simulink library "fdctools"  (Simulink 3.00)
libraries: simulink3 x3
settings Model: LastModifiedBy=Dutchroll

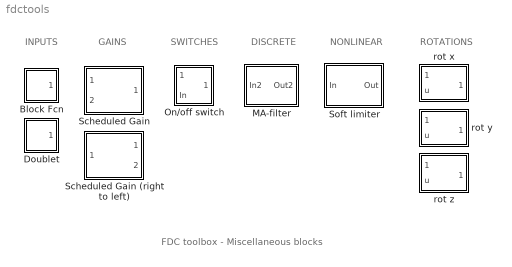
== system fdctools ==
  note: FDC toolbox - Miscellaneous blocks
  note: GAINS
  note: SWITCHES
  note: DISCRETE
  note: NONLINEAR
  note: INPUTS
  note: ROTATIONS
  Block Fcn : Subsystem  mask(Block Fcn){yinit=-1, yblock=2, tstart=1, tstop=4}
      mask prompts: yinit "Initial value (=final value):"; yblock "Amplitude of block (+ = step up, - = step down):"; tstart "Start time of block:"; tstop "Stop time of block:"
      mask help: Block Function
      mask Help:
      | This block implements a block signal.<br><br>
      | Parameters:
      | <li>the initial (=final) value of the signal,
      | <li>the amplitude of the block (positive = upwards, negative = downwards),
      | <li>the start time, and
      | <li>the stop time (which must be later than the start time).
      mask Display: plot(0,0,100,100,[100,60,60,20,20,0],[50,50,89,89,50,50])
  Doublet : Subsystem  mask(Doublet){ts1=1, dt1=1, dt2=1, y1=1, y2=-1, cnst=0}
      mask prompts: ts1 "Start time [sec]:"; dt1 "Length of time interval 1 [sec]:"; dt2 "Length of time interval 2 [sec]:"; cnst "y start (= y final):"
      mask help: Doublet signal.
      mask Help:
      | This block implements a doublet signal:<br><br>
      | y = y1 if  (tstart <= t < tstart+dt1), <br><br>
      | y = y2 if  (tstart+dt1 <= t < tstart+dt1+dt2), <br><br>
      | y = ystart = yfinal if (t < tstart) or (t > tstart+dt1+dt2).<br><br>
      | where tstart is the start time, dt1 is the length of the first time-interval and dt2 is the length of the second time-interval.
      mask Display: plot([0 1 1 2.5 2.5 4 4 5],[0 0 1 1 -1.5 -1.5 0 0])
  MA-filter : Subsystem  mask(Moving Average filter){ns=5, Ts=0.1, uinit=0}
      mask prompts: ns "Number of samples for averaging:"; Ts "Sample time:"; uinit "Initial value of input signal:"
      mask help: Digital Moving Average filter
      mask init:
      | Ama=[zeros(1,ns);[eye(ns-1) zeros(ns-1,1)]]; Bma=[1; zeros(ns-1,1)]; Cma=1/ns*ones(1,ns); Dma=0; xinit=uinit*ones(ns,1);
      mask Help:
      | Digital Moving Average filter.<br><br>
      | y(k) = 1/ns * (u(k) + u(k-1) + ... + u(k-ns)),<br><br>
      | where ns is the number of samples for averaging (to be specified by the user).
      mask Display: disp('Moving\nAverage')
  On/off switch : Subsystem
      mask Type: On/off switch
      mask Description:
      | If input(1) = 1
      |      output = input(2)
      |  else if input(1) = 0
      |      output = 0
      mask Help:
      | On/off switch. If the first input signal is equal to 1, the second input signal will be sent to the output port. Else, if the first input signal is equal to zero, the output signal will be zero.<br><br>
      | 
      | Note: for other values of the first input signal, the resulting output will be unpredictable!
      mask Display: plot(0,0,100,100,[31,31,32,34,34,32,31,31,0],[50,48,47,48,51,53,51,50,50],[100,75,51],[50,50,97]);disp('?')
  Scheduled Gain : Subsystem  mask(Scheduled Gain){K=sin(u[1])}
      mask prompts: K "Gain function:"
      mask help:
      | Inputs: u1 and u2.
      | Output: y.
      |
      | Output equation:   y = K(u1) * u2
      |
      | K is the gain-function, which must be entered below. See the description of the Fcn block from the Nonlinear library for details about valid expressions and the block-characteristics.
      mask init:
      | blockname = [gcb, '/Gain Fcn K(u1)'];
      | set_param(blockname,'Expr',K)
      mask Help:
      | Scheduled Gain function.<br><br>
      | Inputs: u1 and u2, <br><br>
      | output: y, <br><br>
      | output equation:   y = K(u1) * u2.<br><br>
      | K is the gain-function, which must be entered as block-parameter. See the description of the Fcn block from the Nonlinear library for details about valid expressions and the block-characteristics.
      mask Display: plot([0,100,0,0],[0,46,100,0]);disp('K(u1)      ');
  Scheduled Gain (right to left) : Subsystem  Orientation=left  mask(Scheduled Gain){K=sin(u[1])}
      mask prompts: K "Gain function:"
      mask help:
      | Inputs: u1 and u2.
      | Output: y.
      |
      | Output equation:   y = K(u1) * u2
      |
      | K is the gain-function, which must be entered below. See the description of the Fcn block from the Nonlinear library for details about valid expressions and the block-characteristics.
      mask init:
      | blockname = [gcb, '/Gain Fcn K(u1)'];
      | set_param(blockname,'Expr',K)
      mask Help:
      | Scheduled Gain function.<br><br>
      | Inputs: u1 and u2, <br><br>
      | output: y, <br><br>
      | output equation:   y = K(u1) * u2.<br><br>
      | K is the gain-function, which must be entered as block-parameter. See the description of the Fcn block from the Nonlinear library for details about valid expressions and the block-characteristics.
      mask Display: plot([0,-100,0,0],[0,46,100,0]);disp('        K(u1)');
  Soft limiter : Subsystem  mask(Soft limiter){@1=10, @2=10}
      mask prompts: @1 "Limiter range= max. output value= --(min. output value):"; @2 "% of output range where y=u (linear throughput):"
      mask help: Soft limiter with partly linear throughput.
      mask init:
      | max_u=max(@1,1e-16); lin_u=min(0.9999,(max(@2,0)/100))*max_u; uplot=[-5*max_u:0.25*max_u:5*max_u]; for i = 1:length(uplot); yplot(i)=softlim([],[],uplot(i),3,max_u,lin_u); end;
      mask Help:
      | Soft limiter with partly linear throughput. See the source-code of SOFTLIM.M or type HELP SOFTLIM at the command-line to see how this works.<br><br>
      | Parameters:<br><br>
      | <li>Limiter range = maximum output value, which equal <i>minus</i> the minimum output value,
      | <li>percentage of output range where y=u (in this part of the output range the function will yield a linear throughput).
      mask Display: plot(uplot, yplot, max_u*[-5,-1,1,5], max_u*[-1,-1,1,1], 0, -1.3*max_u, 0, 1.2*max_u, max_u*[-5,5], [0,0]);
  rot x : Subsystem
      mask Type: Rotation around X-axis
      mask Description: Direction cosines for rotation around positive X-axis. The first input signal is a (3x1) vector which will be converted to the new reference frame. The second input is a scalar value, which represents the rotation angle.
      mask Help:
      | Direction cosines for rotation around positive X-axis.<br><br>
      | The first input signal is a (3x1) vector which will be converted to the new reference frame. The second input is a scalar value, which represents the rotation angle.
      mask Display: disp('rot x')
  rot y : Subsystem
      mask Type: Rotation around Y-axis
      mask Description: Direction cosines for rotation around positive Y-axis. The first input signal is a (3x1) vector which will be converted to the new reference frame. The second input is a scalar value, which represents the rotation angle.
      mask Help:
      | Direction cosines for rotation around positive Y-axis.<br><br>
      |  The first input signal is a (3x1) vector which will be converted to the new reference frame. The second input is a scalar value, which represents the rotation angle.
      mask Display: disp('rot y')
  rot z : Subsystem
      mask Type: Rotation around Z-axis
      mask Description: Direction cosines for rotation around positive Z-axis. The first input signal is a (3x1) vector which will be converted to the new reference frame. The second input is a scalar value, which represents the rotation angle.
      mask Help:
      | Direction cosines for rotation around positive Z-axis.<br><br>
      | The first input signal is a (3x1) vector which will be converted to the new reference frame. The second input is a scalar value, which represents the rotation angle.
      mask Display: disp('rot z')

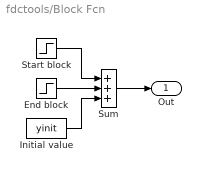
== system fdctools/Block Fcn ==
  End block : Step  Time=tstop  Before=0  After=-yblock  SampleTime=0
  Initial value : Constant  Value=yinit
  Start block : Step  Time=tstart  Before=0  After=yblock  SampleTime=0
  Sum : Sum  Inputs=+++  SaturateOnIntegerOverflow=on
  Out : Outport  Port=1
  wires:
  Initial value/1 -> Sum/3
  Start block/1 -> Sum/1
  End block/1 -> Sum/2
  Sum/1 -> Out/1

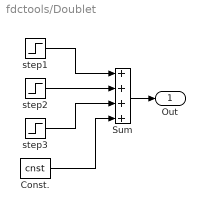
== system fdctools/Doublet ==
  Const. : Constant  Value=cnst
  Sum : Sum  Inputs=++++  SaturateOnIntegerOverflow=on
  step1 : Step  Time=ts1  Before=0  After=y1-cnst  SampleTime=0
  step2 : Step  Time=ts1+dt1  Before=0  After=-y1+y2  SampleTime=0
  step3 : Step  Time=ts1+dt1+dt2  Before=0  After=-y2+cnst  SampleTime=0
  Out : Outport  Port=1
  wires:
  Const./1 -> Sum/4
  step1/1 -> Sum/1
  step2/1 -> Sum/2
  step3/1 -> Sum/3
  Sum/1 -> Out/1

== system fdctools/MA-filter ==
  In2 : Inport  Port=1  PortWidth=-1  SampleTime=-1  DataType=auto
      settings: SignalType=auto
  MA-filter : DiscreteStateSpace  A=Ama  B=Bma  C=Cma  D=Dma  X0=xinit  SampleTime=Ts
  Out2 : Outport  Port=1
  wires:
  In2/1 -> MA-filter/1
  MA-filter/1 -> Out2/1

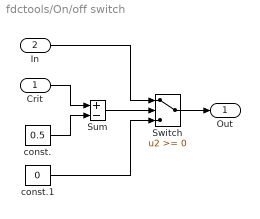
== system fdctools/On/off switch ==
  Crit : Inport  Port=1  PortWidth=-1  SampleTime=-1  DataType=auto
      settings: SignalType=auto
  In : Inport  Port=2  PortWidth=-1  SampleTime=-1  DataType=auto
      settings: SignalType=auto
  Sum : Sum  Inputs=+-  SaturateOnIntegerOverflow=on
  Switch : Switch  Threshold=0
  const. : Constant  Value=0.5
  const.1 : Constant  Value=0
  Out : Outport  Port=1
  wires:
  Crit/1 -> Sum/1
  const.1/1 -> Switch/3
  Sum/1 -> Switch/2
  Switch/1 -> Out/1
  In/1 -> Switch/1
  const./1 -> Sum/2

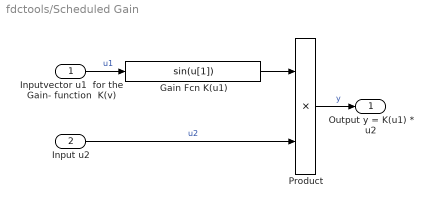
== system fdctools/Scheduled Gain ==
  Inputvector u1  for the Gain- function  K(v) : Inport  Port=1  PortWidth=-1  SampleTime=-1  DataType=auto
      settings: SignalType=auto
  Input u2 : Inport  Port=2  PortWidth=-1  SampleTime=-1  DataType=auto
      settings: SignalType=auto
  Gain Fcn K(u1) : Fcn  Expr=sin(u[1])
  Product : Product  Inputs=2  SaturateOnIntegerOverflow=on
  Output y = K(u1) * u2 : Outport  Port=1
  wires:
  Gain Fcn K(u1)/1 -> Product/1
  Input u2/1 -> Product/2  "u2"
  Product/1 -> Output y = K(u1) * u2/1  "y"
  Inputvector u1  for the Gain- function  K(v)/1 -> Gain Fcn K(u1)/1  "u1"

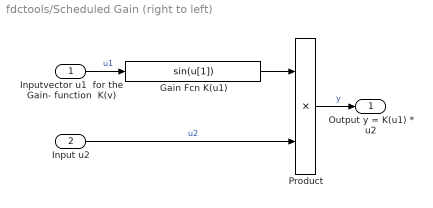
== system fdctools/Scheduled Gain (right to left) ==
  Inputvector u1  for the Gain- function  K(v) : Inport  Port=1  PortWidth=-1  SampleTime=-1  DataType=auto
      settings: SignalType=auto
  Input u2 : Inport  Port=2  PortWidth=-1  SampleTime=-1  DataType=auto
      settings: SignalType=auto
  Gain Fcn K(u1) : Fcn  Expr=sin(u[1])
  Product : Product  Inputs=2  SaturateOnIntegerOverflow=on
  Output y = K(u1) * u2 : Outport  Port=1
  wires:
  Inputvector u1  for the Gain- function  K(v)/1 -> Gain Fcn K(u1)/1  "u1"
  Product/1 -> Output y = K(u1) * u2/1  "y"
  Input u2/1 -> Product/2  "u2"
  Gain Fcn K(u1)/1 -> Product/1

== system fdctools/Soft limiter ==
  In : Inport  Port=1  PortWidth=-1  SampleTime=-1  DataType=auto
      settings: SignalType=auto
  Soft limiter : S-Function  FunctionName=softlim  Parameters=max_u, lin_u  PortCounts=[]  SFunctionModules=''
  Out : Outport  Port=1
  wires:
  In/1 -> Soft limiter/1
  Soft limiter/1 -> Out/1

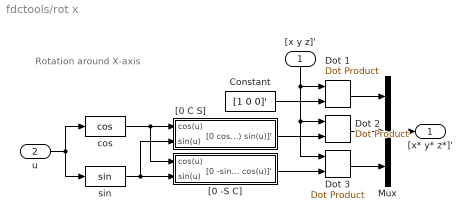
== system fdctools/rot x ==
  note: Rotation around X-axis
  "[x y z]'" : Inport  Orientation=down  Port=1  PortWidth=-1  SampleTime=-1  DataType=auto
      settings: SignalType=auto
  u : Inport  Port=2  PortWidth=-1  SampleTime=-1  DataType=auto
      settings: SignalType=auto
  Constant : Constant  Value=[1 0 0]'
  Dot 1 : simulink3/Math/Dot Product
  Dot 2 : simulink3/Math/Dot Product
  Dot 3 : simulink3/Math/Dot Product
  Mux : Mux  Inputs=3
  "[0 -S C]" : Subsystem
      mask Type: [0 -sin(u) cos(u)]
      mask Display: disp('[0 -sin(u) cos(u)]''');
  "[0 C S]" : Subsystem
      mask Type: [0 cos(u) sin(u)]
      mask Display: disp('[0 cos(u) sin(u)]''');
  cos : Trigonometry  Operator=cos  OutputSignalType=auto
  sin : Trigonometry  Operator=sin  OutputSignalType=auto
  "[x* y* z*]'" : Outport  Port=1
  wires:
  cos/1 -> "[0 C S]"/1(cos(u)), "[0 -S C]"/1(cos(u))
  sin/1 -> "[0 -S C]"/2(sin(u)), "[0 C S]"/2(sin(u))
  Constant/1 -> Dot 1/2
  "[0 C S]"/1("[0 cos(u) sin(u)]'") -> Dot 2/2
  "[0 -S C]"/1("[0 -sin(u) cos(u)]' ") -> Dot 3/2
  "[x y z]'"/1 -> Dot 3/1, Dot 2/1, Dot 1/1
  Dot 1/1 -> Mux/1
  Dot 2/1 -> Mux/2
  Dot 3/1 -> Mux/3
  Mux/1 -> "[x* y* z*]'"/1
  u/1 -> cos/1, sin/1

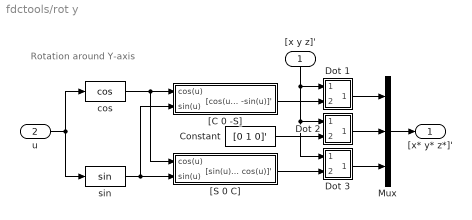
== system fdctools/rot y ==
  note: Rotation around Y-axis
  "[x y z]'" : Inport  Orientation=down  Port=1  PortWidth=-1  SampleTime=-1  DataType=auto
      settings: SignalType=auto
  u : Inport  Port=2  PortWidth=-1  SampleTime=-1  DataType=auto
      settings: SignalType=auto
  Constant : Constant  Value=[0 1 0]'
  Dot 1 : Subsystem  mask(Dot Product){}
      mask help:
      | Inner (dot) product.
      | y=sum(u1.*u2)
      mask init:
      | t=(0:.1:2*pi)';
      | x=cos(t);
      | y=sin(t);
      | r=0.05;
      mask Help: Computes the inner (dot) product of the inputs: sum(u1.*u2).  The inputs are vectors of the same length. Output is a scalar.
      mask Display: patch([x*r+0.5],[y*r+0.5])
  Dot 2 : Subsystem  mask(Dot Product){}
      mask help:
      | Inner (dot) product.
      | y=sum(u1.*u2)
      mask init:
      | t=(0:.1:2*pi)';
      | x=cos(t);
      | y=sin(t);
      | r=0.05;
      mask Help: Computes the inner (dot) product of the inputs: sum(u1.*u2).  The inputs are vectors of the same length. Output is a scalar.
      mask Display: patch([x*r+0.5],[y*r+0.5])
  Dot 3 : Subsystem  mask(Dot Product){}
      mask help:
      | Inner (dot) product.
      | y=sum(u1.*u2)
      mask init:
      | t=(0:.1:2*pi)';
      | x=cos(t);
      | y=sin(t);
      | r=0.05;
      mask Help: Computes the inner (dot) product of the inputs: sum(u1.*u2).  The inputs are vectors of the same length. Output is a scalar.
      mask Display: patch([x*r+0.5],[y*r+0.5])
  Mux : Mux  Inputs=3
  "[C 0 -S]" : Subsystem
      mask Type: [cos(u) 0 -sin(u)]
      mask Display: disp('[cos(u) 0 -sin(u)]''');
  "[S 0 C]" : Subsystem
      mask Type: [sin(u) 0 cos(u)]
      mask Display: disp('[sin(u) 0 cos(u)]''');
  cos : Trigonometry  Operator=cos  OutputSignalType=auto
  sin : Trigonometry  Operator=sin  OutputSignalType=auto
  "[x* y* z*]'" : Outport  Port=1
  wires:
  u/1 -> sin/1, cos/1
  Mux/1 -> "[x* y* z*]'"/1
  Dot 3/1(Out1) -> Mux/3
  Dot 2/1(Out1) -> Mux/2
  Dot 1/1(Out1) -> Mux/1
  "[x y z]'"/1 -> Dot 1/1(In1), Dot 2/1(In1), Dot 3/1(In1)
  "[S 0 C]"/1("[sin(u) 0 cos(u)]' ") -> Dot 3/2(In2)
  sin/1 -> "[C 0 -S]"/2(sin(u)), "[S 0 C]"/2(sin(u))
  cos/1 -> "[S 0 C]"/1(cos(u)), "[C 0 -S]"/1(cos(u))
  Constant/1 -> Dot 2/2(In2)
  "[C 0 -S]"/1("[cos(u) 0 -sin(u)]'") -> Dot 1/2(In2)

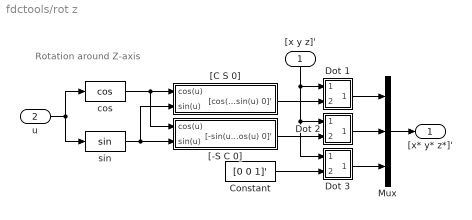
== system fdctools/rot z ==
  note: Rotation around Z-axis
  "[x y z]'" : Inport  Orientation=down  Port=1  PortWidth=-1  SampleTime=-1  DataType=auto
      settings: SignalType=auto
  u : Inport  Port=2  PortWidth=-1  SampleTime=-1  DataType=auto
      settings: SignalType=auto
  Constant : Constant  Value=[0 0 1]'
  Dot 1 : Subsystem  mask(Dot Product){}
      mask help:
      | Inner (dot) product.
      | y=sum(u1.*u2)
      mask init:
      | t=(0:.1:2*pi)';
      | x=cos(t);
      | y=sin(t);
      | r=0.05;
      mask Help: Computes the inner (dot) product of the inputs: sum(u1.*u2).  The inputs are vectors of the same length. Output is a scalar.
      mask Display: patch([x*r+0.5],[y*r+0.5])
  Dot 2 : Subsystem  mask(Dot Product){}
      mask help:
      | Inner (dot) product.
      | y=sum(u1.*u2)
      mask init:
      | t=(0:.1:2*pi)';
      | x=cos(t);
      | y=sin(t);
      | r=0.05;
      mask Help: Computes the inner (dot) product of the inputs: sum(u1.*u2).  The inputs are vectors of the same length. Output is a scalar.
      mask Display: patch([x*r+0.5],[y*r+0.5])
  Dot 3 : Subsystem  mask(Dot Product){}
      mask help:
      | Inner (dot) product.
      | y=sum(u1.*u2)
      mask init:
      | t=(0:.1:2*pi)';
      | x=cos(t);
      | y=sin(t);
      | r=0.05;
      mask Help: Computes the inner (dot) product of the inputs: sum(u1.*u2).  The inputs are vectors of the same length. Output is a scalar.
      mask Display: patch([x*r+0.5],[y*r+0.5])
  Mux : Mux  Inputs=3
  "[-S C 0]" : Subsystem
      mask Type: [-sin(u) cos(u) 0]
      mask Display: disp('[-sin(u) cos(u) 0]''');
  "[C S 0]" : Subsystem
      mask Type: [cos(u) sin(u) 0]
      mask Display: disp('[cos(u) sin(u) 0]''');
  cos : Trigonometry  Operator=cos  OutputSignalType=auto
  sin : Trigonometry  Operator=sin  OutputSignalType=auto
  "[x* y* z*]'" : Outport  Port=1
  wires:
  "[x y z]'"/1 -> Dot 3/1(In1), Dot 2/1(In1), Dot 1/1(In1)
  Dot 1/1(Out1) -> Mux/1
  Dot 2/1(Out1) -> Mux/2
  Dot 3/1(Out1) -> Mux/3
  Mux/1 -> "[x* y* z*]'"/1
  sin/1 -> "[-S C 0]"/2(sin(u)), "[C S 0]"/2(sin(u))
  Constant/1 -> Dot 3/2(In2)
  cos/1 -> "[C S 0]"/1(cos(u)), "[-S C 0]"/1(cos(u))
  u/1 -> cos/1, sin/1
  "[C S 0]"/1("[cos(u) sin(u) 0]'") -> Dot 1/2(In2)
  "[-S C 0]"/1("[-sin(u) cos(u) 0]' ") -> Dot 2/2(In2)

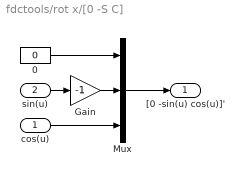
== system fdctools/rot x/[0 -S C] ==
  cos(u) : Inport  Port=1  PortWidth=1  SampleTime=-1  DataType=auto
      settings: SignalType=auto
  sin(u) : Inport  Port=2  PortWidth=1  SampleTime=-1  DataType=auto
      settings: SignalType=auto
  0 : Constant  Value=0
  Gain : Gain  Gain=-1  SaturateOnIntegerOverflow=on
  Mux : Mux  Inputs=3
  "[0 -sin(u) cos(u)]' " : Outport  Port=1
  wires:
  sin(u)/1 -> Gain/1
  Gain/1 -> Mux/2
  Mux/1 -> "[0 -sin(u) cos(u)]' "/1
  0/1 -> Mux/1
  cos(u)/1 -> Mux/3

== system fdctools/rot x/[0 C S] ==
  cos(u) : Inport  Port=1  PortWidth=1  SampleTime=-1  DataType=auto
      settings: SignalType=auto
  sin(u) : Inport  Port=2  PortWidth=1  SampleTime=-1  DataType=auto
      settings: SignalType=auto
  0 : Constant  Value=0
  Mux : Mux  Inputs=3
  "[0 cos(u) sin(u)]'" : Outport  Port=1
  wires:
  sin(u)/1 -> Mux/3
  cos(u)/1 -> Mux/2
  Mux/1 -> "[0 cos(u) sin(u)]'"/1
  0/1 -> Mux/1

== system fdctools/rot y/Dot 1 ==
  In1 : Inport  Port=1  PortWidth=-1  SampleTime=-1  DataType=auto
      settings: SignalType=auto
  In2 : Inport  Port=2  PortWidth=-1  SampleTime=-1  DataType=auto
      settings: SignalType=auto
  S-Function : S-Function  FunctionName=sdotproduct  PortCounts=[]  SFunctionModules=''
  Out1 : Outport  Port=1
  wires:
  S-Function/1 -> Out1/1
  In1/1 -> S-Function/1
  In2/1 -> S-Function/2

== system fdctools/rot y/Dot 2 ==
  In1 : Inport  Port=1  PortWidth=-1  SampleTime=-1  DataType=auto
      settings: SignalType=auto
  In2 : Inport  Port=2  PortWidth=-1  SampleTime=-1  DataType=auto
      settings: SignalType=auto
  S-Function : S-Function  FunctionName=sdotproduct  PortCounts=[]  SFunctionModules=''
  Out1 : Outport  Port=1
  wires:
  S-Function/1 -> Out1/1
  In1/1 -> S-Function/1
  In2/1 -> S-Function/2

== system fdctools/rot y/Dot 3 ==
  In1 : Inport  Port=1  PortWidth=-1  SampleTime=-1  DataType=auto
      settings: SignalType=auto
  In2 : Inport  Port=2  PortWidth=-1  SampleTime=-1  DataType=auto
      settings: SignalType=auto
  S-Function : S-Function  FunctionName=sdotproduct  PortCounts=[]  SFunctionModules=''
  Out1 : Outport  Port=1
  wires:
  S-Function/1 -> Out1/1
  In1/1 -> S-Function/1
  In2/1 -> S-Function/2

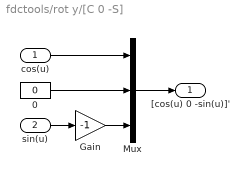
== system fdctools/rot y/[C 0 -S] ==
  cos(u) : Inport  Port=1  PortWidth=1  SampleTime=-1  DataType=auto
      settings: SignalType=auto
  sin(u) : Inport  Port=2  PortWidth=1  SampleTime=-1  DataType=auto
      settings: SignalType=auto
  0 : Constant  Value=0
  Gain : Gain  Gain=-1  SaturateOnIntegerOverflow=on
  Mux : Mux  Inputs=3
  "[cos(u) 0 -sin(u)]'" : Outport  Port=1
  wires:
  sin(u)/1 -> Gain/1
  Gain/1 -> Mux/3
  Mux/1 -> "[cos(u) 0 -sin(u)]'"/1
  cos(u)/1 -> Mux/1
  0/1 -> Mux/2

== system fdctools/rot y/[S 0 C] ==
  cos(u) : Inport  Port=1  PortWidth=1  SampleTime=-1  DataType=auto
      settings: SignalType=auto
  sin(u) : Inport  Port=2  PortWidth=1  SampleTime=-1  DataType=auto
      settings: SignalType=auto
  0 : Constant  Value=0
  Mux : Mux  Inputs=3
  "[sin(u) 0 cos(u)]' " : Outport  Port=1
  wires:
  sin(u)/1 -> Mux/1
  cos(u)/1 -> Mux/3
  Mux/1 -> "[sin(u) 0 cos(u)]' "/1
  0/1 -> Mux/2

== system fdctools/rot z/Dot 1 ==
  In1 : Inport  Port=1  PortWidth=-1  SampleTime=-1  DataType=auto
      settings: SignalType=auto
  In2 : Inport  Port=2  PortWidth=-1  SampleTime=-1  DataType=auto
      settings: SignalType=auto
  S-Function : S-Function  FunctionName=sdotproduct  PortCounts=[]  SFunctionModules=''
  Out1 : Outport  Port=1
  wires:
  S-Function/1 -> Out1/1
  In1/1 -> S-Function/1
  In2/1 -> S-Function/2

== system fdctools/rot z/Dot 2 ==
  In1 : Inport  Port=1  PortWidth=-1  SampleTime=-1  DataType=auto
      settings: SignalType=auto
  In2 : Inport  Port=2  PortWidth=-1  SampleTime=-1  DataType=auto
      settings: SignalType=auto
  S-Function : S-Function  FunctionName=sdotproduct  PortCounts=[]  SFunctionModules=''
  Out1 : Outport  Port=1
  wires:
  S-Function/1 -> Out1/1
  In1/1 -> S-Function/1
  In2/1 -> S-Function/2

== system fdctools/rot z/Dot 3 ==
  In1 : Inport  Port=1  PortWidth=-1  SampleTime=-1  DataType=auto
      settings: SignalType=auto
  In2 : Inport  Port=2  PortWidth=-1  SampleTime=-1  DataType=auto
      settings: SignalType=auto
  S-Function : S-Function  FunctionName=sdotproduct  PortCounts=[]  SFunctionModules=''
  Out1 : Outport  Port=1
  wires:
  S-Function/1 -> Out1/1
  In1/1 -> S-Function/1
  In2/1 -> S-Function/2

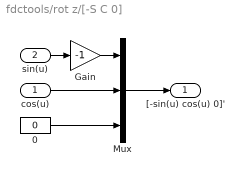
== system fdctools/rot z/[-S C 0] ==
  cos(u) : Inport  Port=1  PortWidth=1  SampleTime=-1  DataType=auto
      settings: SignalType=auto
  sin(u) : Inport  Port=2  PortWidth=1  SampleTime=-1  DataType=auto
      settings: SignalType=auto
  0 : Constant  Value=0
  Gain : Gain  Gain=-1  SaturateOnIntegerOverflow=on
  Mux : Mux  Inputs=3
  "[-sin(u) cos(u) 0]' " : Outport  Port=1
  wires:
  cos(u)/1 -> Mux/2
  sin(u)/1 -> Gain/1
  0/1 -> Mux/3
  Gain/1 -> Mux/1
  Mux/1 -> "[-sin(u) cos(u) 0]' "/1

== system fdctools/rot z/[C S 0] ==
  cos(u) : Inport  Port=1  PortWidth=1  SampleTime=-1  DataType=auto
      settings: SignalType=auto
  sin(u) : Inport  Port=2  PortWidth=1  SampleTime=-1  DataType=auto
      settings: SignalType=auto
  0 : Constant  Value=0
  Mux : Mux  Inputs=3
  "[cos(u) sin(u) 0]'" : Outport  Port=1
  wires:
  0/1 -> Mux/3
  sin(u)/1 -> Mux/2
  cos(u)/1 -> Mux/1
  Mux/1 -> "[cos(u) sin(u) 0]'"/1
